simulink model "task6_3"  (R2016b)
settings: Solver=VariableStepAuto  StartTime=0.0  StopTime=10.0  RelTol=1e-3
settings Model: Creator=Suvansh  LastModifiedBy=Suvansh

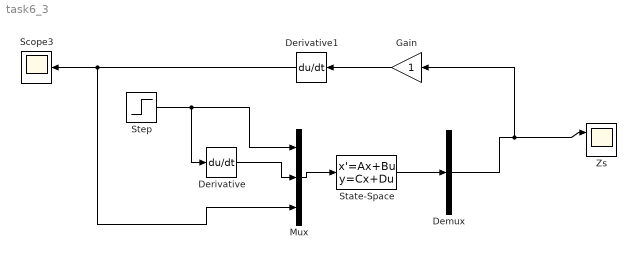
== system task6_3 ==
  Demux : Demux  Outputs=1
  Derivative : Derivative
  Derivative1 : Derivative
  Gain : Gain
  Mux : Mux  Inputs=3
  Scope3 : Scope
  State-Space : StateSpace  A=|  B=|  C=[1 0 0 0];  D=[0 0 0 ] ;  X0=0
      A=|
      | [0 1 0 0; 
      |     -ks/ms  0  ks/ms  0;
      |     0 0 0 1 ;
      |     ks/mp 0 (-ks-kp)/mp -cp1;];
      B=|
      | [  0  0 0 ;1/ms  0 0 ; 
      | 0 0 0;
      |   1/mp  kp/mp -cp1/mp ;];
  Step : Step  After=0.05  SampleTime=0
  Zs : Scope  NumInputPorts=2
  wires:
  Mux/1 -> State-Space/1
  Step/1 -> Mux/1, Derivative/1
  State-Space/1 -> Demux/1
  Demux/1 -> Gain/1, Zs/1
  Derivative/1 -> Mux/2
  Derivative1/1 -> Mux/3, Scope3/1
  Gain/1 -> Derivative1/1
